simulink subsystem "BAM_Controller"  (R2026a)
settings: Solver=VariableStepAuto
undefined symbols (not defined in the file): DiscIntNeverNeededParam, SimIn, SimPar
libraries: simulink x11, starslibMathOperations x2, sharedTrackingLibrary x1, simulink_extras x1, starslibAxisTransformations x1
(part 1 of 3)
settings Model: Creator=macheson  LastModifiedBy=wyatt

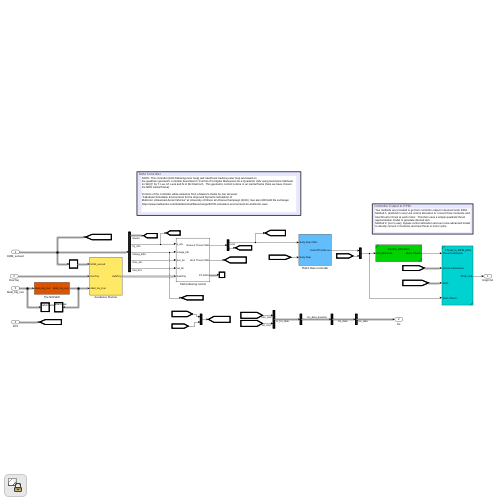
[thumbnail: Simulink's stored preview of the top-level diagram]
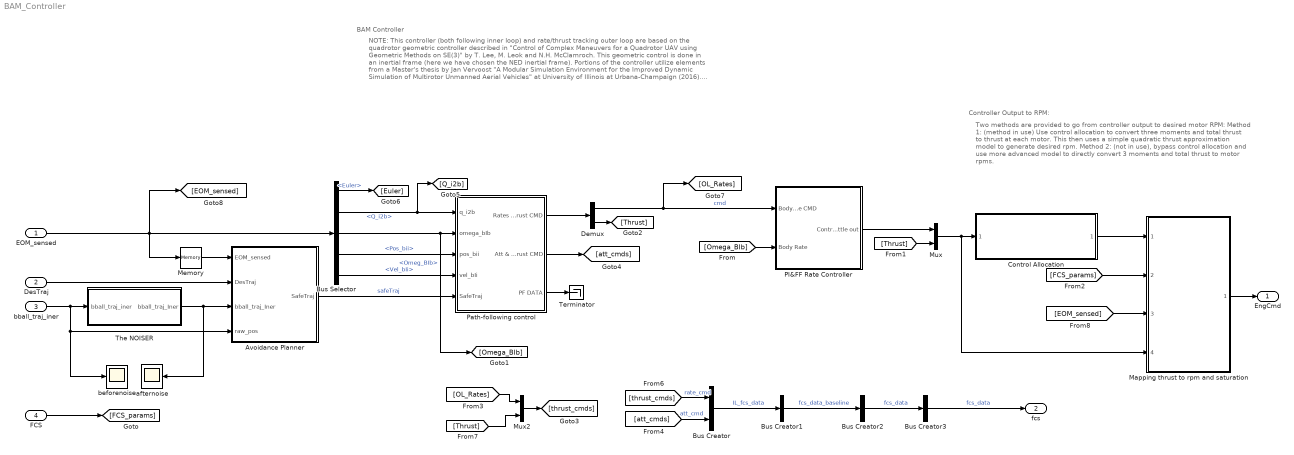
== system BAM_Controller ==
  note: NOTE: This controller (both following inner loop) and rate/thrust tracking outer loop are based on
      | the quadrotor geometric controller described in "Control of Complex Maneuvers for a Quadrotor UAV using Geometric Methods on SE(3)" by T. Lee, M. Leok and N.H. McClamroch. This geometric control is done in an inertial frame (here we have chosen the NED inertial frame).
      |
      | Portions of the controller utilize elements from a Master's thesis by Jan Vervoost
      | "A Modular Simulation Environment for the Improved Dynamic Simulation of
      | Multirotor Unmanned Aerial Vehicles" at University of Illinois at Urbana-Champaign (2016). See also MATLAB file exchange:
      | https://www.mathworks.com/matlabcentral/fileexchange/59705-simulation-environment-for-multirotor-uavs
  note: BAM Controller
  note: Controller Output to RPM:
  note: Two methods are provided to go from controller output to desired motor RPM:
      | Method 1: (method in use) Use control allocation to convert three moments and total thrust to thrust at each motor. This then uses a simple quadratic thrust approximation model to generate desired rpm.
      | Method 2: (not in use), bypass control allocation and use more advanced model to directly convert 3 moments and total thrust to motor rpms.
  EOM_sensed : Inport
  DesTraj : Inport  Port=2
  bball_traj_iner : Inport  Port=3
  FCS : Inport  Port=4
  Avoidance Planner : Subsystem
  Bus Creator : BusCreator  Inputs=2
  Bus Creator1 : BusCreator  Inputs=1
  Bus Creator2 : BusCreator  Inputs=1
  Bus Creator3 : BusCreator  Inputs=1
  Bus Selector : BusSelector  OutputSignals=WorldRelativeData.Euler,InertialData.Q_i2b,InertialData.Omeg_BIb,InertialData.Pos_bii,InertialData.Vel_bIi
  Control Allocation : Subsystem  ReferencedSubsystem=Control_Allocation
  Demux : Demux  Outputs=[3 1]
  Mapping thrust to rpm and saturation : Subsystem  ReferencedSubsystem=Thrust_to_RPM_MDL
  Memory : Memory
  Mux : Mux  Inputs=2
  Mux2 : Mux  Inputs=2
  PI&FF Rate Controller : Subsystem
  Path-following control : Subsystem
  Terminator : Terminator
  The NOISER : Subsystem
  afternoise : Scope
      settings: ActiveDisplayYMinimum=-1  ActiveDisplayYMaximum=1  DataLoggingVariableName=ScopeData14
  beforenoise : Scope
      settings: ActiveDisplayYMinimum=-48.7860252359001  ActiveDisplayYMaximum=146.64274370042804  DataLoggingVariableName=ScopeData15
  EngCmd : Outport  VectorParamsAs1DForOutWhenUnconnected=off
  fcs : Outport  Port=2  VectorParamsAs1DForOutWhenUnconnected=off
  wires:
  Path-following control/1(Rates & Thrust CMD) -> Demux/1
  [FCS_params] -> Mapping thrust to rpm and saturation/2
  Path-following control/3(PF DATA) -> Terminator/1
  EOM_sensed/1 -> [EOM_sensed], Bus Selector/1, Memory/1
  FCS/1 -> [FCS_params]
  PI&FF Rate Controller/1(Control/Throttle out) -> Mux/1
  Bus Selector/2 -> Path-following control/1(q_i2b), [Q_i2b]  "<Q_i2b>"
  Bus Selector/5 -> Path-following control/4(vel_bIi)  "<Vel_bIi>"
  Bus Selector/4 -> Path-following control/3(pos_bii)  "<Pos_bii>"
  Bus Selector/3 -> Path-following control/2(omega_bIb), [Omega_BIb]  "<Omeg_BIb>"
  [Omega_BIb] -> PI&FF Rate Controller/2(Body Rate)
  Demux/2 -> [Thrust]
  Demux/1 -> PI&FF Rate Controller/1(Body Rate CMD), [OL_Rates]  "cmd"
  DesTraj/1 -> Avoidance Planner/2(DesTraj)
  Bus Creator/1 -> Bus Creator1/1  "IL_fcs_data"
  Bus Creator1/1 -> Bus Creator2/1  "fcs_data_baseline"
  Bus Creator2/1 -> Bus Creator3/1  "fcs_data"
  Bus Creator3/1 -> fcs/1  "fcs_data"
  Path-following control/2(Att & Thrust CMD) -> [att_cmds]
  Bus Selector/1 -> [Euler]  "<Euler>"
  [thrust_cmds] -> Bus Creator/1  "rate_cmd"
  Mux2/1 -> [thrust_cmds]
  [OL_Rates] -> Mux2/1
  [Thrust] -> Mux2/2
  [Thrust] -> Mux/2
  Mux/1 -> Control Allocation/1, Mapping thrust to rpm and saturation/4
  Mapping thrust to rpm and saturation/1 -> EngCmd/1
  [att_cmds] -> Bus Creator/2  "att_cmd"
  [EOM_sensed] -> Mapping thrust to rpm and saturation/3
  Control Allocation/1 -> Mapping thrust to rpm and saturation/1
  Avoidance Planner/1(SafeTraj) -> Path-following control/5(SafeTraj)  "safeTraj"
  Memory/1 -> Avoidance Planner/1(EOM_sensed)
  bball_traj_iner/1 -> The NOISER/1(bball_traj_iner), Avoidance Planner/4(raw_pos), beforenoise/1
  The NOISER/1(bball_traj_Iner) -> Avoidance Planner/3(bball_traj_Iner), afternoise/1

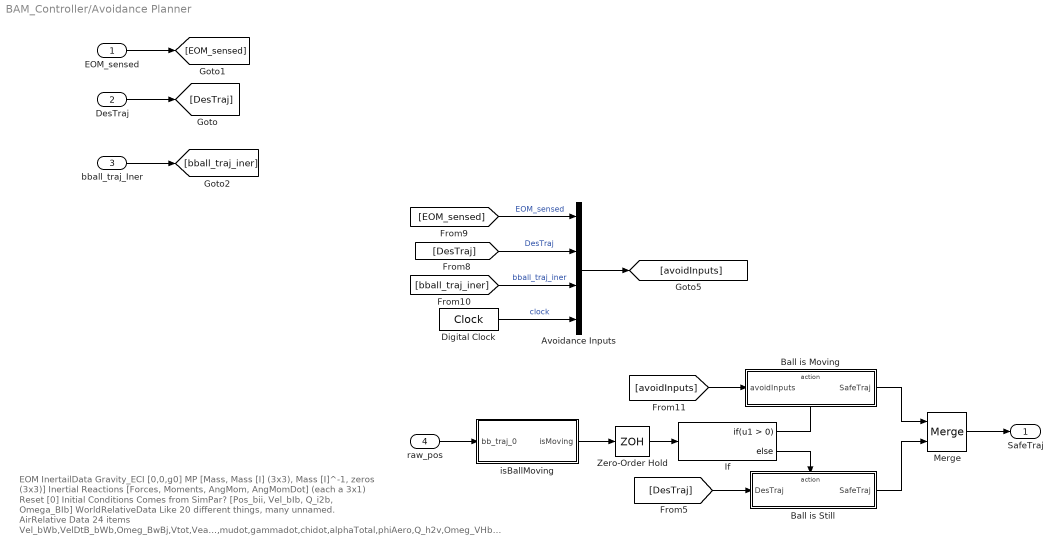
== system BAM_Controller/Avoidance Planner ==
  note: EOM
      | InertailData
      | Gravity_ECI
      | [0,0,g0]
      | MP
      | [Mass, Mass [I] (3x3), Mass [I]^-1, zeros (3x3)]
      | Inertial Reactions
      | [Forces, Moments, AngMom, AngMomDot] (each a 3x1)
      | Reset [0]
      | Initial Conditions
      | Comes from SimPar?
      | [Pos_bii, Vel_bIb, Q_i2b, Omega_BIb]
      | WorldRelativeData
      | Like 20 different things, many unnamed.
      | AirRelative Data
      | 24 items
      | Vel_bWb,VelDtB_bWb,Omeg_BwBj,Vtot,Veas,Vcas,Mach,qbar,qc,alpha,beta,mu,gamma,chi,Vtotdot,alphadot,betadot,mudot,gammadot,chidot,alphaTotal,phiAero,Q_h2v,Omeg_VHb
      | WRD is built using Env and ID, ARD is buid from Env and WRD
      | Traj_Iner = DesTraj (Designated Trajectory)
      | SimPar.RefInputs.trajectory
      | [wptVect, timeVect, parseVect]
      | Bball_traj
      | [pos_i, vel_i, acc_i, chi_des, chi_dot_des, time_violate_flag]
      | [(3,1), (3,1), (3,1), 1, 1, 1]
  EOM_sensed : Inport
  DesTraj : Inport  Port=2
  bball_traj_Iner : Inport  Port=3
  raw_pos : Inport  Port=4
  Avoidance Inputs : BusCreator  Inputs=4
  Ball is Moving : Subsystem  TreatAsAtomicUnit=on
  Ball is Still : Subsystem  TreatAsAtomicUnit=on
  Digital Clock : DigitalClock  SampleTime=.005
  If : If
  Merge : Merge
  Zero-Order Hold : ZeroOrderHold  SampleTime=.005
  isBallMoving : Subsystem
  SafeTraj : Outport
  wires:
  Digital Clock/1 -> Avoidance Inputs/4  "clock"
  isBallMoving/1(isMoving) -> Zero-Order Hold/1
  Avoidance Inputs/1 -> [avoidInputs]
  [bball_traj_iner] -> Avoidance Inputs/3  "bball_traj_iner"
  [DesTraj] -> Avoidance Inputs/2  "DesTraj"
  [EOM_sensed] -> Avoidance Inputs/1  "EOM_sensed"
  bball_traj_Iner/1 -> [bball_traj_iner]
  EOM_sensed/1 -> [EOM_sensed]
  DesTraj/1 -> [DesTraj]
  If/1 -> Ball is Moving/Action
  [avoidInputs] -> Ball is Moving/1(avoidInputs)
  Zero-Order Hold/1 -> If/1
  Ball is Moving/1(SafeTraj) -> Merge/1
  [DesTraj] -> Ball is Still/1(DesTraj)
  raw_pos/1 -> isBallMoving/1(bb_traj_0)
  If/2 -> Ball is Still/Action
  Merge/1 -> SafeTraj/1
  Ball is Still/1(SafeTraj) -> Merge/2

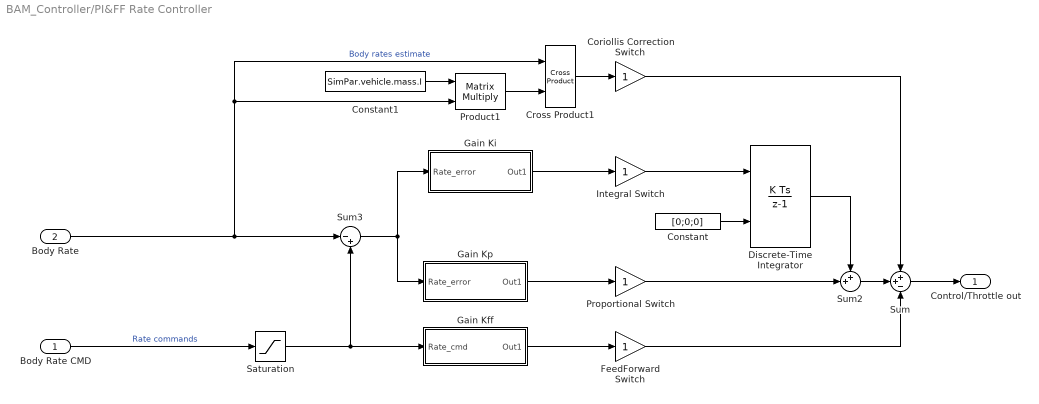
== system BAM_Controller/PI&FF Rate Controller ==
  Body Rate CMD : Inport
  Body Rate : Inport  Port=2
  Constant : Constant  Value=[0;0;0]  VectorParams1D=off
  Constant1 : Constant  Value=SimPar.vehicle.mass.I
  Coriollis Correction Switch : Gain
  Cross Product1 : starslibMathOperations/Cross Product
  Discrete-Time Integrator : DiscreteIntegrator  InitialConditionSource=external  SampleTime=SimIn.FCS.t_control  LimitOutput=on  UpperSaturationLimit=0.05  LowerSaturationLimit=-0.05  ICPrevOutput=DiscIntNeverNeededParam  ICPrevScaledInput=DiscIntNeverNeededParam
  FeedForward Switch : Gain
  Gain Kff : Subsystem
  Gain Ki : Subsystem
  Gain Kp : Subsystem
  Integral Switch : Gain
  Product1 : Product  Multiplication=Matrix(*)  RndMeth=Zero
  Proportional Switch : Gain
  Saturation : Saturate  UpperLimit=SimIn.FCS.maxRateCmd(3)  LowerLimit=-SimIn.FCS.maxRateCmd(3)
  Sum : Sum  Inputs=++-
  Sum2 : Sum  Inputs=++|
  Sum3 : Sum  Inputs=|-+
  Control/Throttle out : Outport  VectorParamsAs1DForOutWhenUnconnected=off
  wires:
  Coriollis Correction Switch/1 -> Sum/1
  Cross Product1/1 -> Coriollis Correction Switch/1
  Body Rate/1 -> Sum3/1, Product1/2, Cross Product1/1  "Body rates estimate"
  Constant1/1 -> Product1/1
  Product1/1 -> Cross Product1/2
  FeedForward Switch/1 -> Sum/3
  Proportional Switch/1 -> Sum2/2
  Integral Switch/1 -> Discrete-Time Integrator/1
  Constant/1 -> Discrete-Time Integrator/2
  Gain Ki/1(Out1) -> Integral Switch/1
  Saturation/1 -> Sum3/2, Gain Kff/1(Rate_cmd)
  Gain Kff/1(Out1) -> FeedForward Switch/1
  Sum2/1 -> Sum/2
  Sum3/1 -> Gain Kp/1(Rate_error), Gain Ki/1(Rate_error)
  Body Rate CMD/1 -> Saturation/1  "Rate commands"
  Sum/1 -> Control/Throttle out/1
  Gain Kp/1(Out1) -> Proportional Switch/1
  Discrete-Time Integrator/1 -> Sum2/1

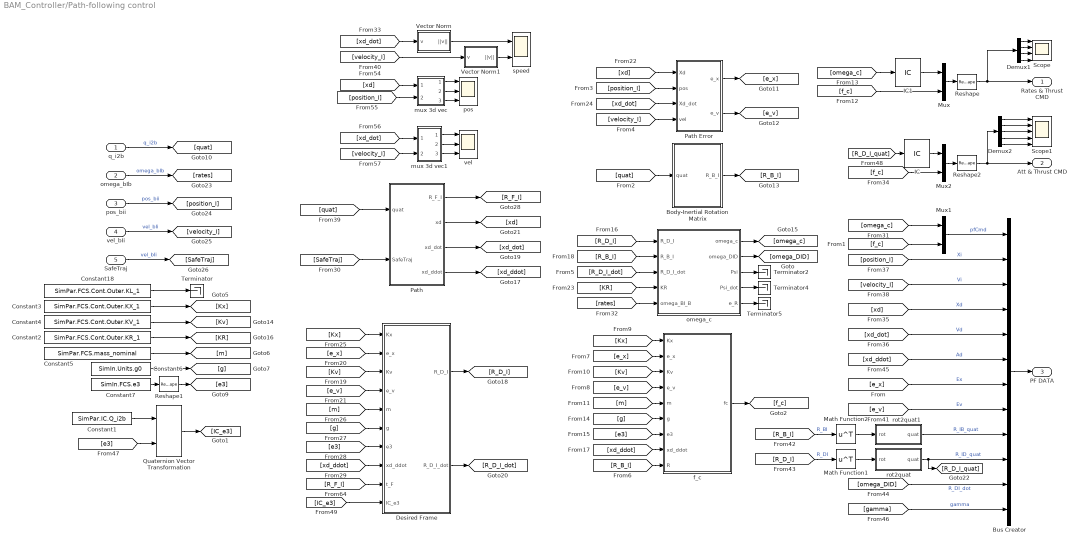
== system BAM_Controller/Path-following control ==
  q_i2b : Inport
  omega_bIb : Inport  Port=2
  pos_bii : Inport  Port=3
  vel_bIi : Inport  Port=4
  SafeTraj : Inport  Port=5
  Body-Inertial Rotation Matrix : Subsystem
  Bus Creator : BusCreator  Inputs=12
  Constant1 : Constant  Value=SimPar.IC.Q_i2b  VectorParams1D=off
  Constant18 : Constant  Value=SimPar.FCS.Cont.Outer.KL_1
  Constant2 : Constant  Value=SimPar.FCS.Cont.Outer.KR_1
  Constant3 : Constant  Value=SimPar.FCS.Cont.Outer.KX_1
  Constant4 : Constant  Value=SimPar.FCS.Cont.Outer.KV_1
  Constant5 : Constant  Value=SimPar.FCS.mass_nominal
  Constant6 : Constant  Value=SimIn.Units.g0
  Constant7 : Constant  Value=SimIn.FCS.e3  VectorParams1D=off
  Demux1 : Demux
  Demux2 : Demux  Outputs=5
  Desired Frame : Subsystem
  IC : InitialCondition  Value=SimIn.IC.Q_i2b
  IC1 : InitialCondition  Value=SimIn.IC.Omega_BIb
  Math Function1 : Math  Operator=transpose  SignedPower=on
  Math Function2 : Math  Operator=transpose  SignedPower=on
  Mux : Mux  Inputs=2
  Mux1 : Mux  Inputs=2
  Mux2 : Mux  Inputs=2
  Path : Subsystem
  Path Error : Subsystem
  Quaternion Vector Transformation : starslibAxisTransformations/Quaternion Vector Transformation  n=0
  Reshape : Reshape  OutputDimensionality=Column vector (2-D)
  Reshape1 : Reshape  OutputDimensionality=Column vector (2-D)
  Reshape2 : Reshape  OutputDimensionality=Column vector (2-D)
  Scope : Scope  NumInputPorts=4
      settings: SampleTime=SimIn.model_params.sim_rate  ActiveDisplayYMinimum=-0.00169  ActiveDisplayYMaximum=0.00216
  Scope1 : Scope  NumInputPorts=5
      settings: SampleTime=SimIn.model_params.sim_rate  ActiveDisplayYMinimum=-0.00169  ActiveDisplayYMaximum=0.00216
  Terminator{,2,4..5} (4 alike) : Terminator
  Vector Norm : Subsystem  mask(Vector Norm){}
      mask help: Calculates the 2-norm of the input vector.
      settings: CopyFcn=set_param(gcb,'LinkStatus','none')
  Vector Norm1 : Subsystem  mask(Vector Norm){}
      mask help: Calculates the 2-norm of the input vector.
      settings: CopyFcn=set_param(gcb,'LinkStatus','none')
  f_c : Subsystem
  mux 3d vec : Subsystem
  mux 3d vec1 : Subsystem
  omega_c : Subsystem
  pos : Scope  NumInputPorts=3
      settings: SampleTime=SimIn.model_params.sim_rate  ActiveDisplayYMinimum=-7386.0314  ActiveDisplayYMaximum=820.67244  DataLoggingVariableName=ScopeData2
  rot2quat : Subsystem  mask(RotationMatrix2Quat){}
      mask help: Rotation matrix to quaternion conversion.
      settings: CopyFcn=set_param(gcb,'LinkStatus','none')
  rot2quat1 : Subsystem  mask(RotationMatrix2Quat){}
      mask help: Rotation matrix to quaternion conversion.
      settings: CopyFcn=set_param(gcb,'LinkStatus','none')
  speed : Scope  NumInputPorts=2
      settings: SampleTime=SimIn.model_params.sim_rate  ActiveDisplayYMinimum=-0.50184  ActiveDisplayYMaximum=4.51655
  vel : Scope  NumInputPorts=3
      settings: SampleTime=SimIn.model_params.sim_rate  ActiveDisplayYMinimum=-3E-12  ActiveDisplayYMaximum=2.5E-11  DataLoggingVariableName=ScopeData3
  Rates & Thrust CMD : Outport  VectorParamsAs1DForOutWhenUnconnected=off
  Att & Thrust CMD : Outport  Port=2  VectorParamsAs1DForOutWhenUnconnected=off
  PF DATA : Outport  Port=3  VectorParamsAs1DForOutWhenUnconnected=off
  wires:
  IC/1 -> Mux2/1
  IC1/1 -> Mux/1
  [omega_c] -> IC1/1
  [R_D_I_quat] -> IC/1
  Demux2/5 -> Scope1/5
  [f_c] -> Mux2/2
  Demux2/2 -> Scope1/2
  Demux2/4 -> Scope1/4
  Reshape2/1 -> Demux2/1, Att & Thrust CMD/1
  Mux2/1 -> Reshape2/1
  Demux2/3 -> Scope1/3
  Demux2/1 -> Scope1/1
  [SafeTraj] -> Path/2(SafeTraj)
  SafeTraj/1 -> [SafeTraj]  "vel_bIi"
  vel_bIi/1 -> [velocity_I]  "vel_bIi"
  pos_bii/1 -> [position_I]  "pos_bii"
  omega_bIb/1 -> [rates]  "omega_bIb"
  [velocity_I] -> Vector Norm1/1(v)
  Vector Norm1/1(||v||) -> speed/2
  Vector Norm/1(||v||) -> speed/1
  [xd_dot] -> Vector Norm/1(v)
  rot2quat1/1(quat) -> Bus Creator/9  "R_IB_quat"
  Math Function2/1 -> rot2quat1/1(rot)
  omega_c/2(omega_DID) -> [omega_DID]
  [R_D_I] -> Math Function1/1  "R_DI"
  Math Function1/1 -> rot2quat/1(rot)
  Bus Creator/1 -> PF DATA/1
  [gamma] -> Bus Creator/12  "gamma"
  [omega_DID] -> Bus Creator/11  "R_DI_dot"
  rot2quat/1(quat) -> Bus Creator/10, [R_D_I_quat]  "R_ID_quat"
  [R_B_I] -> Math Function2/1  "R_BI"
  [e_v] -> Bus Creator/8  "Ev"
  [e_x] -> Bus Creator/7  "Ex"
  [xd_ddot] -> Bus Creator/6  "Ad"
  [xd_dot] -> Bus Creator/5  "Vd"
  [xd] -> Bus Creator/4  "Xd"
  [velocity_I] -> Bus Creator/3  "Vi"
  [position_I] -> Bus Creator/2  "Xi"
  [omega_c] -> Mux1/1
  Mux1/1 -> Bus Creator/1  "pfCmd"
  [f_c] -> Mux1/2
  [quat] -> Path/1(quat)
  f_c/1(fc) -> [f_c]
  [R_B_I] -> f_c/9(R)
  [xd_ddot] -> f_c/8(xd_ddot)
  [e3] -> f_c/7(e3)
  [g] -> f_c/6(g)
  [m] -> f_c/5(m)
  [e_v] -> f_c/4(e_v)
  [Kv] -> f_c/3(Kv)
  [e_x] -> f_c/2(e_x)
  [Kx] -> f_c/1(Kx)
  omega_c/1(omega_c) -> [omega_c]
  omega_c/5(e_R) -> Terminator5/1
  omega_c/4(Psi_dot) -> Terminator4/1
  omega_c/3(Psi) -> Terminator2/1
  [rates] -> omega_c/5(omega_BI_B)
  [KR] -> omega_c/4(KR)
  [R_D_I_dot] -> omega_c/3(R_D_I_dot)
  [R_B_I] -> omega_c/2(R_B_I)
  [R_D_I] -> omega_c/1(R_D_I)
  Desired Frame/2(R_D_I_dot) -> [R_D_I_dot]
  Desired Frame/1(R_D_I) -> [R_D_I]
  Path/1(R_F_I) -> [R_F_I]
  Path/4(xd_ddot) -> [xd_ddot]
  Path/3(xd_dot) -> [xd_dot]
  Path/2(xd) -> [xd]
  [velocity_I] -> mux 3d vec1/2(In2)
  [xd_dot] -> mux 3d vec1/1(In1)
  mux 3d vec1/3(Out3) -> vel/3
  mux 3d vec1/2(Out2) -> vel/2
  mux 3d vec1/1(Out1) -> vel/1
  [position_I] -> mux 3d vec/2(In2)
  [xd] -> mux 3d vec/1(In1)
  mux 3d vec/3(Out3) -> pos/3
  mux 3d vec/2(Out2) -> pos/2
  mux 3d vec/1(Out1) -> pos/1
  Reshape1/1 -> [e3]
  Constant6/1 -> [g]
  Constant5/1 -> [m]
  Constant7/1 -> Reshape1/1
  Constant2/1 -> [KR]
  Constant4/1 -> [Kv]
  Constant3/1 -> [Kx]
  Constant18/1 -> Terminator/1
  Body-Inertial Rotation Matrix/1(R_B_I) -> [R_B_I]
  [quat] -> Body-Inertial Rotation Matrix/1(quat)
  Reshape/1 -> Demux1/1, Rates & Thrust CMD/1
  Demux1/4 -> Scope/4
  Demux1/3 -> Scope/3
  Demux1/2 -> Scope/2
  Demux1/1 -> Scope/1
  Mux/1 -> Reshape/1
  [f_c] -> Mux/2
  [xd_dot] -> Path Error/3(Xd_dot)
  [xd] -> Path Error/1(Xd)
  Path Error/2(e_v) -> [e_v]
  Path Error/1(e_x) -> [e_x]
  [velocity_I] -> Path Error/4(vel)
  [position_I] -> Path Error/2(pos)
  q_i2b/1 -> [quat]  "q_i2b"
  [Kx] -> Desired Frame/1(Kx)
  [e_x] -> Desired Frame/2(e_x)
  [Kv] -> Desired Frame/3(Kv)
  [e_v] -> Desired Frame/4(e_v)
  [m] -> Desired Frame/5(m)
  [g] -> Desired Frame/6(g)
  [e3] -> Desired Frame/7(e3)
  [xd_ddot] -> Desired Frame/8(xd_ddot)
  [R_F_I] -> Desired Frame/9(t_F)
  Constant1/1 -> Quaternion Vector Transformation/1
  [IC_e3] -> Desired Frame/10(IC_e3)
  [e3] -> Quaternion Vector Transformation/2
  Quaternion Vector Transformation/1 -> [IC_e3]

== system BAM_Controller/The NOISER ==
  note: 0 = no noise
      | 0.1 = 10% noise
      | 0.5 = 50% noise
  bball_traj_iner : Inport
  Band-Limited White Noise : simulink/Sources/Band-Limited White Noise  Cov=[0]  Ts=0.1  seed=[23341]
  Bus Creator : BusCreator  Inputs=6  OutDataTypeStr=Bus: BUS_REF_INPUT_INER
  Bus Selector1 : BusSelector  OutputSignals=pos_i,vel_i,acc_i,chi_des,chi_dot_des,time_violate_flag
  Sum5 : Sum  Inputs=++|
  bball_traj_Iner : Outport
  wires:
  Band-Limited White Noise/1 -> Sum5/1
  Bus Selector1/1 -> Sum5/2  "<pos_i>"
  Bus Creator/1 -> bball_traj_Iner/1
  Sum5/1 -> Bus Creator/1  "pos_i"
  Bus Selector1/2 -> Bus Creator/2  "<vel_i>"
  Bus Selector1/3 -> Bus Creator/3  "<acc_i>"
  Bus Selector1/4 -> Bus Creator/4  "<chi_des>"
  Bus Selector1/5 -> Bus Creator/5  "<chi_dot_des>"
  Bus Selector1/6 -> Bus Creator/6  "<time_violate_flag>"
  bball_traj_iner/1 -> Bus Selector1/1

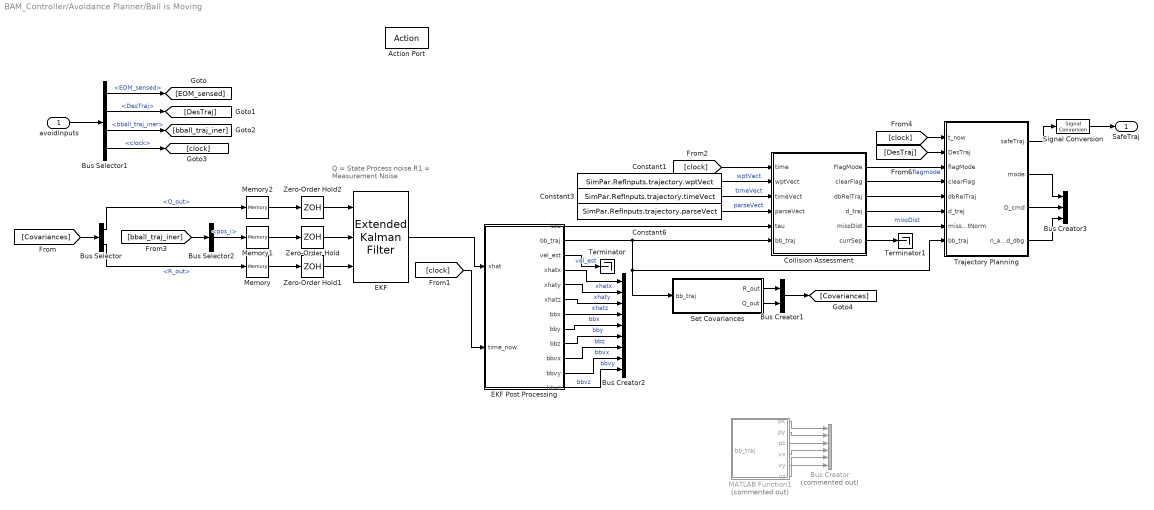
== system BAM_Controller/Avoidance Planner/Ball is Moving ==
  note: Q = State Process noise
      | R1 = Measurement Noise
  avoidInputs : Inport
  Action Port : ActionPort
  Bus Creator : BusCreator  Commented=on  Inputs=6
  Bus Creator1 : BusCreator  Inputs=2
  Bus Creator2 : BusCreator  Inputs=9
  Bus Creator3 : BusCreator  Inputs=3
  Bus Selector : BusSelector  OutputSignals=Q_out,R_out
  Bus Selector1 : BusSelector  OutputSignals=EOM_sensed,DesTraj,bball_traj_iner,clock
  Bus Selector2 : BusSelector  OutputSignals=pos_i
  Collision Assessment : MATLAB Function  TreatAsAtomicUnit=on
  Constant1 : Constant  Value=SimPar.RefInputs.trajectory.wptVect
  Constant3 : Constant  Value=SimPar.RefInputs.trajectory.timeVect
  Constant6 : Constant  Value=SimPar.RefInputs.trajectory.parseVect
  EKF : sharedTrackingLibrary/Extended Kalman Filter  StateTransitionFcn=ballStateTransitionFcn  HasStateTransitionJacobianFcn=off  HasAdditiveProcessNoise=Additive  ProcessNoise=diag([0.01 0.01 0.01 0.1 0.1 0.1])  HasTimeVaryingProcessNoise=on  HasStateTransitionFcnExtraArgument=0  InitialState=[-4.55720896517794 90.7482900530603 -0.440339408827839 19.065442307483 8.77448054331578 -23.8809138575693]  InitialStateCovariance=diag([0, 0, 0, 0, 0, 0])  MeasurementFcn1=ballMeasurementFcn  HasMeasurementJacobianFcn1=off  HasMeasurementEnablePort1=off  HasAdditiveMeasurementNoise1=Additive  MeasurementNoise1=diag([0.1 0.1 0.1])  HasTimeVaryingMeasurementNoise1=on  HasMeasurementFcnExtraArgument1=0  HasMeasurementWrapping1=off  HasMeasurementJacobianFcn2=off  HasMeasurementEnablePort2=off  HasAdditiveMeasurementNoise2=Additive  MeasurementNoise2=1  HasTimeVaryingMeasurementNoise2=off  HasMeasurementFcnExtraArgument2=0  HasMeasurementWrapping2=off  HasMeasurementJacobianFcn3=off  HasMeasurementEnablePort3=off  HasAdditiveMeasurementNoise3=Additive  MeasurementNoise3=1  HasTimeVaryingMeasurementNoise3=off  HasMeasurementFcnExtraArgument3=0  HasMeasurementWrapping3=off  HasMeasurementJacobianFcn4=off  HasMeasurementEnablePort4=off  HasAdditiveMeasurementNoise4=Additive  MeasurementNoise4=1  HasTimeVaryingMeasurementNoise4=off  HasMeasurementFcnExtraArgument4=0  HasMeasurementWrapping4=off  HasMeasurementJacobianFcn5=off  HasMeasurementEnablePort5=off  HasAdditiveMeasurementNoise5=Additive  MeasurementNoise5=1  HasTimeVaryingMeasurementNoise5=off  HasMeasurementFcnExtraArgument5=0  HasMeasurementWrapping5=off  EnableMultirate=off  StateTransitionFcnSampleTime=1  MeasurementFcn1SampleTime=1  MeasurementFcn2SampleTime=1  MeasurementFcn3SampleTime=1  MeasurementFcn4SampleTime=1  MeasurementFcn5SampleTime=1  UseCurrentEstimator=on  OutputStateCovariance=off  DataType=double  SampleTime=.005  NumberOfMeasurements=1
  EKF Post Processing : MATLAB Function  TreatAsAtomicUnit=on
  MATLAB Function1 : MATLAB Function  Commented=on  TreatAsAtomicUnit=on
  Memory : Memory  InheritSampleTime=on
  Memory1 : Memory  InheritSampleTime=on
  Memory2 : Memory  InheritSampleTime=on
  Set Covariances : MATLAB Function  TreatAsAtomicUnit=on
  Signal Conversion : SignalConversion  ConversionOutput=Virtual bus  OverrideOpt=off
  Terminator : Terminator
  Terminator1 : Terminator
  Trajectory Planning : MATLAB Function  TreatAsAtomicUnit=on
  Zero-Order Hold : ZeroOrderHold  SampleTime=.005
  Zero-Order Hold1 : ZeroOrderHold  SampleTime=.005
  Zero-Order Hold2 : ZeroOrderHold  SampleTime=.005
  SafeTraj : Outport
  wires:
  Collision Assessment/6(currSep) -> Terminator1/1
  Trajectory Planning/4(n_avoid_dbg) -> Bus Creator3/3
  Trajectory Planning/3(D_cmd) -> Bus Creator3/2
  Trajectory Planning/2(mode) -> Bus Creator3/1
  Collision Assessment/4(d_traj) -> Trajectory Planning/6(d_traj)
  [clock] -> Trajectory Planning/1(t_now)
  [clock] -> Collision Assessment/1(time)
  EKF Post Processing/12(bbvz) -> Bus Creator2/9  "bbvz"
  EKF Post Processing/4(xhatx) -> Bus Creator2/1  "xhatx"
  EKF Post Processing/5(xhaty) -> Bus Creator2/2  "xhaty"
  EKF Post Processing/6(xhatz) -> Bus Creator2/3  "xhatz"
  EKF Post Processing/7(bbx) -> Bus Creator2/4  "bbx"
  EKF Post Processing/8(bby) -> Bus Creator2/5  "bby"
  EKF Post Processing/9(bbz) -> Bus Creator2/6  "bbz"
  EKF Post Processing/10(bbvx) -> Bus Creator2/7  "bbvx"
  EKF Post Processing/11(bbvy) -> Bus Creator2/8  "bbvy"
  EKF Post Processing/3(vel_est) -> Terminator/1  "vel_est"
  Bus Selector1/4 -> [clock]  "<clock>"
  [clock] -> EKF Post Processing/2(time_now)
  MATLAB Function1/6(vz) -> Bus Creator/6
  MATLAB Function1/5(vy) -> Bus Creator/5
  MATLAB Function1/4(vx) -> Bus Creator/4
  MATLAB Function1/3(pz) -> Bus Creator/3
  MATLAB Function1/2(py) -> Bus Creator/2
  MATLAB Function1/1(px) -> Bus Creator/1
  Set Covariances/2(Q_out) -> Bus Creator1/2
  Set Covariances/1(R_out) -> Bus Creator1/1
  Signal Conversion/1 -> SafeTraj/1
  Bus Selector2/1 -> Memory1/1  "<pos_i>"
  [bball_traj_iner] -> Bus Selector2/1
  Bus Selector1/3 -> [bball_traj_iner]  "<bball_traj_iner>"
  Bus Selector1/2 -> [DesTraj]  "<DesTraj>"
  Bus Selector1/1 -> [EOM_sensed]  "<EOM_sensed>"
  avoidInputs/1 -> Bus Selector1/1
  Bus Selector/2 -> Memory/1  "<R_out>"
  [Covariances] -> Bus Selector/1
  Bus Creator1/1 -> [Covariances]
  EKF/1 -> EKF Post Processing/1(xhat)
  Zero-Order Hold/1 -> EKF/2
  Memory2/1 -> Zero-Order Hold2/1
  Bus Selector/1 -> Memory2/1  "<Q_out>"
  Zero-Order Hold2/1 -> EKF/1
  Zero-Order Hold1/1 -> EKF/3
  Memory/1 -> Zero-Order Hold1/1
  Memory1/1 -> Zero-Order Hold/1
  Trajectory Planning/1(safeTraj) -> Signal Conversion/1
  [DesTraj] -> Trajectory Planning/2(DesTraj)
  Collision Assessment/2(clearFlag) -> Trajectory Planning/4(clearFlag)
  Constant3/1 -> Collision Assessment/3(timeVect)  "timeVect"
  Collision Assessment/5(missDist) -> Trajectory Planning/7(missDistNorm)  "missDist"
  Collision Assessment/3(dbRelTraj) -> Trajectory Planning/5(dbRelTraj)
  EKF Post Processing/2(bb_traj) -> Collision Assessment/6(bb_traj), Trajectory Planning/8(bb_traj), Set Covariances/1(bb_traj)
  EKF Post Processing/1(tau) -> Collision Assessment/5(tau)
  Constant1/1 -> Collision Assessment/2(wptVect)  "wptVect"
  Collision Assessment/1(FlagMode) -> Trajectory Planning/3(flagMode)  "flagmode"
  Constant6/1 -> Collision Assessment/4(parseVect)  "parseVect"

== system BAM_Controller/Avoidance Planner/Ball is Still ==
  DesTraj : Inport
  Action Port : ActionPort
  SafeTraj : Outport
  wires:
  DesTraj/1 -> SafeTraj/1

== system BAM_Controller/Avoidance Planner/isBallMoving ==
  bb_traj_0 : Inport
  Bus Selector : BusSelector  OutputSignals=pos_i
  Compare To Constant : simulink/Logic and Bit Operations/Compare To Constant  relop=>  const=0.01  OutDataTypeStr=boolean
  Compare To Constant1 : simulink/Logic and Bit Operations/Compare To Constant  relop=>  const=0.01  OutDataTypeStr=boolean
  Constant7 : Constant  Value=1e-9
  Constant8 : Constant  Value=0
  Data Type Conversion2 : DataTypeConversion  OutDataTypeStr=boolean  SaturateOnIntegerOverflow=off  RndMeth=Floor
  Data Type Conversion3 : DataTypeConversion  OutDataTypeStr=boolean  SaturateOnIntegerOverflow=off  RndMeth=Floor
  Dot Product1 : DotProduct  OutDataTypeStr=Inherit: Inherit via internal rule
  S-R Flip-Flop1 : simulink_extras/Flip Flops/S-R Flip-Flop  initial_condition=0
  Sqrt1 : Sqrt
  Sum2 : Sum  Inputs=|+-
  Sum3 : Sum  Inputs=|++
  Unit Delay1 : UnitDelay  SampleTime=-1
  Zero-Order Hold2 : ZeroOrderHold  SampleTime=.005
  isMoving : Outport
  wires:
  Compare To Constant/1 -> Zero-Order Hold2/1
  Sqrt1/1 -> Compare To Constant/1
  Bus Selector/1 -> Unit Delay1/1, Sum2/1  "<pos_i>"
  bb_traj_0/1 -> Bus Selector/1
  Zero-Order Hold2/1 -> isMoving/1
  Sum3/1 -> Sqrt1/1
  Dot Product1/1 -> Sum3/1
  Unit Delay1/1 -> Sum2/2
  Sum2/1 -> Dot Product1/1, Dot Product1/2
  Constant8/1 -> Data Type Conversion3/1
  Constant7/1 -> Sum3/2
  Data Type Conversion3/1 -> S-R Flip-Flop1/2
  Data Type Conversion2/1 -> S-R Flip-Flop1/1
  Compare To Constant1/1 -> Data Type Conversion2/1

== system BAM_Controller/PI&FF Rate Controller/Gain Kff ==
  Rate_cmd : Inport
  Constant : Constant  Value=SimPar.vehicle.mass.I
  Constant1 : Constant  Value=SimPar.FCS.Cont.Inner.Kff_1
  Diagonalize Vector : Subsystem
  Product : Product  Multiplication=Matrix(*)  RndMeth=Zero
  Product1 : Product  Multiplication=Matrix(*)  RndMeth=Zero
  Out1 : Outport  VectorParamsAs1DForOutWhenUnconnected=off
  wires:
  Diagonalize Vector/1(Matrix) -> Product1/2
  Constant/1 -> Product1/1
  Product/1 -> Out1/1
  Constant1/1 -> Diagonalize Vector/1(Vector)
  Rate_cmd/1 -> Product/2
  Product1/1 -> Product/1

== system BAM_Controller/PI&FF Rate Controller/Gain Ki ==
  Rate_error : Inport
  Constant : Constant  Value=SimPar.vehicle.mass.I
  Constant1 : Constant  Value=SimPar.FCS.Cont.Inner.Ki_1
  Diagonalize Vector : Subsystem
  Product : Product  Multiplication=Matrix(*)  RndMeth=Zero
  Product1 : Product  Multiplication=Matrix(*)  RndMeth=Zero
  Out1 : Outport  VectorParamsAs1DForOutWhenUnconnected=off
  wires:
  Diagonalize Vector/1(Matrix) -> Product1/2
  Constant/1 -> Product1/1
  Product/1 -> Out1/1
  Constant1/1 -> Diagonalize Vector/1(Vector)
  Rate_error/1 -> Product/2
  Product1/1 -> Product/1

== system BAM_Controller/PI&FF Rate Controller/Gain Kp ==
  Rate_error : Inport
  Constant : Constant  Value=SimPar.vehicle.mass.I
  Constant1 : Constant  Value=SimPar.FCS.Cont.Inner.Kp_1
  Diagonalize Vector : Subsystem
  Product : Product  Multiplication=Matrix(*)  RndMeth=Zero
  Product1 : Product  Multiplication=Matrix(*)  RndMeth=Zero
  Out1 : Outport  VectorParamsAs1DForOutWhenUnconnected=off
  wires:
  Diagonalize Vector/1(Matrix) -> Product1/2
  Constant1/1 -> Diagonalize Vector/1(Vector)
  Constant/1 -> Product1/1
  Product/1 -> Out1/1
  Rate_error/1 -> Product/2
  Product1/1 -> Product/1

== system BAM_Controller/Path-following control/Body-Inertial Rotation Matrix ==
  quat : Inport
  MATLAB Function : MATLAB Function  TreatAsAtomicUnit=on
  Math Function6 : Math  Operator=transpose  SignedPower=on
  R_B_I : Outport  VectorParamsAs1DForOutWhenUnconnected=off
  wires:
  quat/1 -> MATLAB Function/1(q)
  MATLAB Function/1(R) -> Math Function6/1
  Math Function6/1 -> R_B_I/1

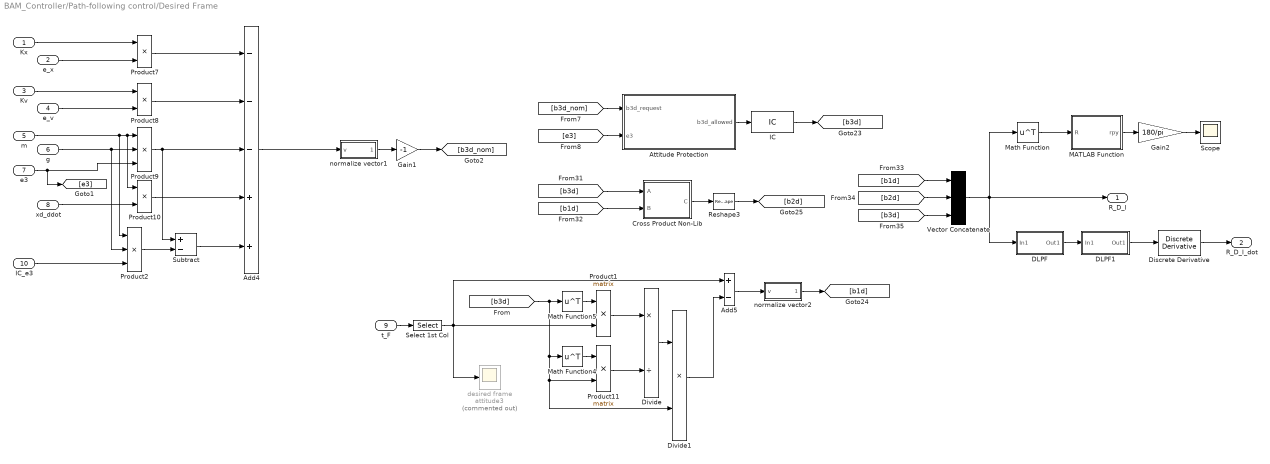
== system BAM_Controller/Path-following control/Desired Frame ==
  Kx : Inport
  e_x : Inport  Port=2
  Kv : Inport  Port=3
  e_v : Inport  Port=4
  m : Inport  Port=5
  g : Inport  Port=6
  e3 : Inport  Port=7
  xd_ddot : Inport  Port=8
  t_F : Inport  Port=9
  IC_e3 : Inport  Port=10
  Add4 : Sum  Inputs=---++
  Add5 : Sum  Inputs=+-
  Attitude Protection : Subsystem
  Cross Product Non-Lib : Subsystem
  DLPF : Subsystem  mask{w=20}
      mask prompts: w "Bandwidth"
      mask Display:
      | fprintf('%d rps',w)
      | port_label('input',  1, 'u')
      | port_label('output', 1, 'uf')
  DLPF1 : Subsystem  mask{w=20}
      mask prompts: w "Bandwidth"
      mask Display:
      | fprintf('%d rps',w)
      | port_label('input',  1, 'u')
      | port_label('output', 1, 'uf')
  Discrete Derivative : simulink/Discrete/Discrete Derivative  gainval=1.0  ICPrevScaledInput=0.0  OutMin=[]  OutMax=[]  OutDataType=fixdt(1, 16)  OutScaling=2^-10  DoSatur=off
  Divide : Product  Inputs=*/
  Divide1 : Product  Inputs=**
  Gain1 : Gain  Gain=-1
  Gain2 : Gain  Gain=180/pi
  IC : InitialCondition  Value=[0;0;1]
  MATLAB Function : MATLAB Function  TreatAsAtomicUnit=on
  Math Function : Math  Operator=transpose  SignedPower=on
  Math Function4 : Math  Operator=transpose  SignedPower=on
  Math Function5 : Math  Operator=transpose  SignedPower=on
  Product1 : Product  Multiplication=Matrix(*)
  Product10 : Product
  Product11 : Product  Multiplication=Matrix(*)
  Product2 : Product  Inputs=3
  Product7 : Product
  Product8 : Product
  Product9 : Product  Inputs=3
  Reshape3 : Reshape  OutputDimensionality=Column vector (2-D)
  Scope : Scope
  Select 1st Col : Selector  NumberOfDimensions=2  InputPortWidth=3  IndexOptions=Select all,Index vector (dialog)  Indices=[1 3],1  OutputSizes=1,1
  Subtract : Sum  Inputs=+-
  Vector Concatenate : Concatenate  NumInputs=3  Mode=Multidimensional array  ConcatenateDimension=2
  desired frame attitude3 : Scope  Commented=on
      settings: SampleTime=FCS.t_control  ActiveDisplayYMinimum=-0.67068  ActiveDisplayYMaximum=1.18563  DataLoggingVariableName=ScopeData2
  normalize vector1 : Subsystem
  normalize vector2 : Subsystem
  R_D_I : Outport  VectorParamsAs1DForOutWhenUnconnected=off
  R_D_I_dot : Outport  Port=2  VectorParamsAs1DForOutWhenUnconnected=off
  wires:
  Math Function/1 -> MATLAB Function/1(R)
  IC/1 -> [b3d]
  normalize vector2/1(v / ||v||) -> [b1d]
  Select 1st Col/1 -> Product1/2, Add5/1, desired frame attitude3/1
  Vector Concatenate/1 -> DLPF/1(In1), R_D_I/1, Math Function/1
  Attitude Protection/1(b3d_allowed) -> IC/1
  [e3] -> Attitude Protection/2(e3)
  [b3d_nom] -> Attitude Protection/1(b3d_request)
  Gain2/1 -> Scope/1
  MATLAB Function/1(rpy) -> Gain2/1
  DLPF1/1(Out1) -> Discrete Derivative/1
  DLPF/1(Out1) -> DLPF1/1(In1)
  Discrete Derivative/1 -> R_D_I_dot/1
  Product11/1 -> Divide/2
  Math Function5/1 -> Product1/1
  Divide/1 -> Divide1/1
  Divide1/1 -> Add5/2
  Product1/1 -> Divide/1
  Math Function4/1 -> Product11/1
  [b3d] -> Math Function5/1, Math Function4/1, Product11/2, Divide1/2
  t_F/1 -> Select 1st Col/1
  [b1d] -> Vector Concatenate/1
  [b3d] -> Vector Concatenate/3
  Cross Product Non-Lib/1(C) -> Reshape3/1
  [b1d] -> Cross Product Non-Lib/2(B)
  [b2d] -> Vector Concatenate/2
  [b3d] -> Cross Product Non-Lib/1(A)
  Reshape3/1 -> [b2d]
  Add5/1 -> normalize vector2/1(v)
  normalize vector1/1(v / ||v||) -> Gain1/1
  Add4/1 -> normalize vector1/1(v)
  Gain1/1 -> [b3d_nom]
  xd_ddot/1 -> Product10/2
  IC_e3/1 -> Product2/3
  Product2/1 -> Subtract/2
  e_x/1 -> Product7/2
  e3/1 -> [e3], Product9/3
  Product7/1 -> Add4/1
  Product9/1 -> Add4/3, Subtract/1
  Kv/1 -> Product8/1
  e_v/1 -> Product8/2
  Product10/1 -> Add4/4
  Kx/1 -> Product7/1
  m/1 -> Product9/1, Product10/1, Product2/1
  Subtract/1 -> Add4/5
  g/1 -> Product2/2, Product9/2
  Product8/1 -> Add4/2

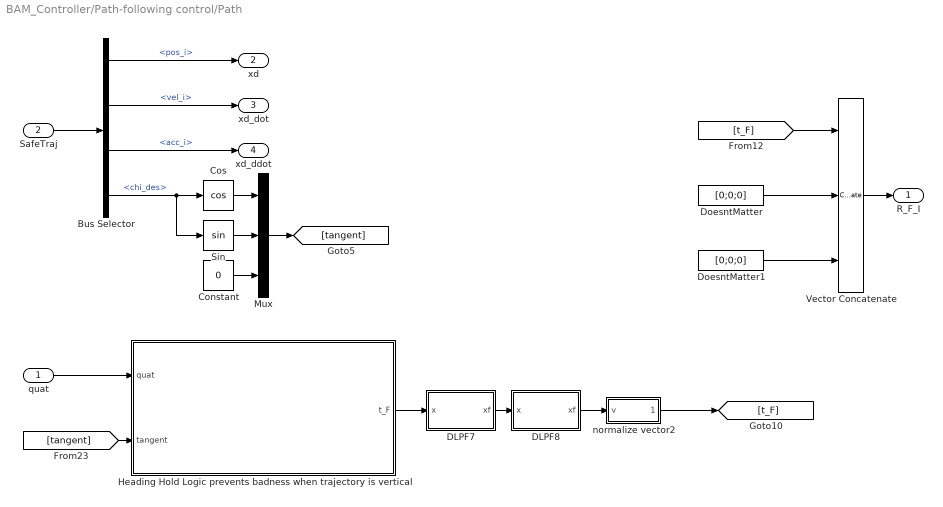
== system BAM_Controller/Path-following control/Path ==
  quat : Inport
  SafeTraj : Inport  Port=2
  Bus Selector : BusSelector  OutputSignals=pos_i,vel_i,acc_i,chi_des
  Constant : Constant  Value=0
  Cos : Trigonometry  Operator=cos
  DLPF7 : Subsystem  mask(Discrete Low-Pass Filter){bw=0.5}
      mask prompts: bw "Bandwidth"
      mask help: Low pass filter a signal with a discrete integrator. Initial condition is obtained from input.
      mask init:
      | set_param(gcb,'LinkStatus','none')
      settings: CopyFcn=set_param(gcb,'LinkStatus','none')
      mask Display:
      | port_label('input',1,'x');
      | port_label('output',1,'xf');
      | 
      | disp([get_param(gcb,'bw') ' rad/s']);
  DLPF8 : Subsystem  mask(Discrete Low-Pass Filter){bw=0.5}
      mask prompts: bw "Bandwidth"
      mask help: Low pass filter a signal with a discrete integrator. Initial condition is obtained from input.
      mask init:
      | set_param(gcb,'LinkStatus','none')
      settings: CopyFcn=set_param(gcb,'LinkStatus','none')
      mask Display:
      | port_label('input',1,'x');
      | port_label('output',1,'xf');
      | 
      | disp([get_param(gcb,'bw') ' rad/s']);
  DoesntMatter : Constant  Value=[0;0;0]  VectorParams1D=off
  DoesntMatter1 : Constant  Value=[0;0;0]  VectorParams1D=off
  Heading Hold Logic prevents badness when trajectory is vertical : Subsystem
  Mux : Mux  Inputs=3
  Sin : Trigonometry
  Vector Concatenate : Concatenate  NumInputs=3  Mode=Multidimensional array  ConcatenateDimension=2
  normalize vector2 : Subsystem
  R_F_I : Outport  VectorParamsAs1DForOutWhenUnconnected=off
  xd : Outport  Port=2  VectorParamsAs1DForOutWhenUnconnected=off
  xd_dot : Outport  Port=3  VectorParamsAs1DForOutWhenUnconnected=off
  xd_ddot : Outport  Port=4  VectorParamsAs1DForOutWhenUnconnected=off
  wires:
  Constant/1 -> Mux/3
  Sin/1 -> Mux/2
  Cos/1 -> Mux/1
  Bus Selector/4 -> Cos/1, Sin/1  "<chi_des>"
  Bus Selector/3 -> xd_ddot/1  "<acc_i>"
  Bus Selector/2 -> xd_dot/1  "<vel_i>"
  Bus Selector/1 -> xd/1  "<pos_i>"
  SafeTraj/1 -> Bus Selector/1
  normalize vector2/1(v / ||v||) -> [t_F]
  DLPF8/1(xf) -> normalize vector2/1(v)
  DLPF7/1(xf) -> DLPF8/1(x)
  Heading Hold Logic prevents badness when trajectory is vertical/1(t_F) -> DLPF7/1(x)
  [tangent] -> Heading Hold Logic prevents badness when trajectory is vertical/2(tangent)
  quat/1 -> Heading Hold Logic prevents badness when trajectory is vertical/1(quat)
  DoesntMatter1/1 -> Vector Concatenate/3
  DoesntMatter/1 -> Vector Concatenate/2
  Mux/1 -> [tangent]
  Vector Concatenate/1 -> R_F_I/1
  [t_F] -> Vector Concatenate/1

== system BAM_Controller/Path-following control/Path Error ==
  Xd : Inport
  pos : Inport  Port=2
  Xd_dot : Inport  Port=3
  vel : Inport  Port=4
  Add : Sum  Inputs=+-
  Add1 : Sum  Inputs=+-
  e_x : Outport  VectorParamsAs1DForOutWhenUnconnected=off
  e_v : Outport  Port=2  VectorParamsAs1DForOutWhenUnconnected=off
  wires:
  Xd_dot/1 -> Add1/2
  Xd/1 -> Add/2
  Add1/1 -> e_v/1
  Add/1 -> e_x/1
  pos/1 -> Add/1
  vel/1 -> Add1/1

== system BAM_Controller/Path-following control/Vector Norm ==
  v : Inport
  Math Function1 : Math  Operator=transpose  SignedPower=on
  Matrix Multiply1 : Product  Multiplication=Matrix(*)
  Reshape7 : Reshape  OutputDimensionality=Column vector (2-D)
  Sqrt3 : Sqrt
  ||v|| : Outport  VectorParamsAs1DForOutWhenUnconnected=off
  wires:
  Sqrt3/1 -> ||v||/1
  v/1 -> Reshape7/1
  Math Function1/1 -> Matrix Multiply1/1
  Matrix Multiply1/1 -> Sqrt3/1
  Reshape7/1 -> Matrix Multiply1/2, Math Function1/1

== system BAM_Controller/Path-following control/Vector Norm1 ==
  v : Inport
  Math Function1 : Math  Operator=transpose  SignedPower=on
  Matrix Multiply1 : Product  Multiplication=Matrix(*)
  Reshape7 : Reshape  OutputDimensionality=Column vector (2-D)
  Sqrt3 : Sqrt
  ||v|| : Outport  VectorParamsAs1DForOutWhenUnconnected=off
  wires:
  Reshape7/1 -> Math Function1/1, Matrix Multiply1/2
  Matrix Multiply1/1 -> Sqrt3/1
  Math Function1/1 -> Matrix Multiply1/1
  v/1 -> Reshape7/1
  Sqrt3/1 -> ||v||/1

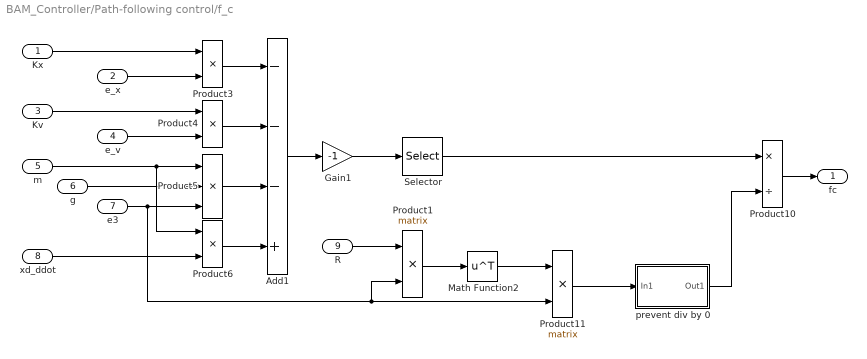
== system BAM_Controller/Path-following control/f_c ==
  Kx : Inport
  e_x : Inport  Port=2
  Kv : Inport  Port=3
  e_v : Inport  Port=4
  m : Inport  Port=5
  g : Inport  Port=6
  e3 : Inport  Port=7
  xd_ddot : Inport  Port=8
  R : Inport  Port=9
  Add1 : Sum  Inputs=---+
  Gain1 : Gain  Gain=-1
  Math Function2 : Math  Operator=transpose  SignedPower=on
  Product1 : Product  Multiplication=Matrix(*)
  Product10 : Product  Inputs=*/
  Product11 : Product  Multiplication=Matrix(*)
  Product3 : Product
  Product4 : Product
  Product5 : Product  Inputs=3
  Product6 : Product
  Selector : Selector  InputPortWidth=3  IndexOptions=Index vector (dialog)  Indices=[3]  OutputSizes=1
  prevent div by 0 : Subsystem
  fc : Outport  VectorParamsAs1DForOutWhenUnconnected=off
  wires:
  prevent div by 0/1(Out1) -> Product10/2
  Product11/1 -> prevent div by 0/1(In1)
  Selector/1 -> Product10/1
  Gain1/1 -> Selector/1
  Product10/1 -> fc/1
  Math Function2/1 -> Product11/1
  Add1/1 -> Gain1/1
  R/1 -> Product1/1
  e_x/1 -> Product3/2
  e_v/1 -> Product4/2
  e3/1 -> Product1/2, Product11/2, Product5/3
  Product1/1 -> Math Function2/1
  Kx/1 -> Product3/1
  Kv/1 -> Product4/1
  Product5/1 -> Add1/3
  Product3/1 -> Add1/1
  xd_ddot/1 -> Product6/2
  m/1 -> Product5/1, Product6/1
  Product6/1 -> Add1/4
  Product4/1 -> Add1/2
  g/1 -> Product5/2

== system BAM_Controller/Path-following control/mux 3d vec ==
  In1 : Inport
  In2 : Inport  Port=2
  Demux2 : Demux  Outputs=3
  Demux3 : Demux  Outputs=3
  Mux4 : Mux  Inputs=2
  Mux5 : Mux  Inputs=2
  Mux6 : Mux  Inputs=2
  Out1 : Outport  VectorParamsAs1DForOutWhenUnconnected=off
  Out2 : Outport  Port=2  VectorParamsAs1DForOutWhenUnconnected=off
  Out3 : Outport  Port=3  VectorParamsAs1DForOutWhenUnconnected=off
  wires:
  Demux2/2 -> Mux5/1
  Demux2/3 -> Mux6/1
  In1/1 -> Demux2/1
  In2/1 -> Demux3/1
  Mux6/1 -> Out3/1
  Mux5/1 -> Out2/1
  Mux4/1 -> Out1/1
  Demux3/3 -> Mux6/2
  Demux3/1 -> Mux4/2
  Demux3/2 -> Mux5/2
  Demux2/1 -> Mux4/1

== system BAM_Controller/Path-following control/mux 3d vec1 ==
  In1 : Inport
  In2 : Inport  Port=2
  Demux2 : Demux  Outputs=3
  Demux3 : Demux  Outputs=3
  Mux4 : Mux  Inputs=2
  Mux5 : Mux  Inputs=2
  Mux6 : Mux  Inputs=2
  Out1 : Outport  VectorParamsAs1DForOutWhenUnconnected=off
  Out2 : Outport  Port=2  VectorParamsAs1DForOutWhenUnconnected=off
  Out3 : Outport  Port=3  VectorParamsAs1DForOutWhenUnconnected=off
  wires:
  Demux2/1 -> Mux4/1
  Demux3/2 -> Mux5/2
  Demux3/1 -> Mux4/2
  Demux3/3 -> Mux6/2
  Mux4/1 -> Out1/1
  Mux5/1 -> Out2/1
  Mux6/1 -> Out3/1
  In2/1 -> Demux3/1
  In1/1 -> Demux2/1
  Demux2/3 -> Mux6/1
  Demux2/2 -> Mux5/1

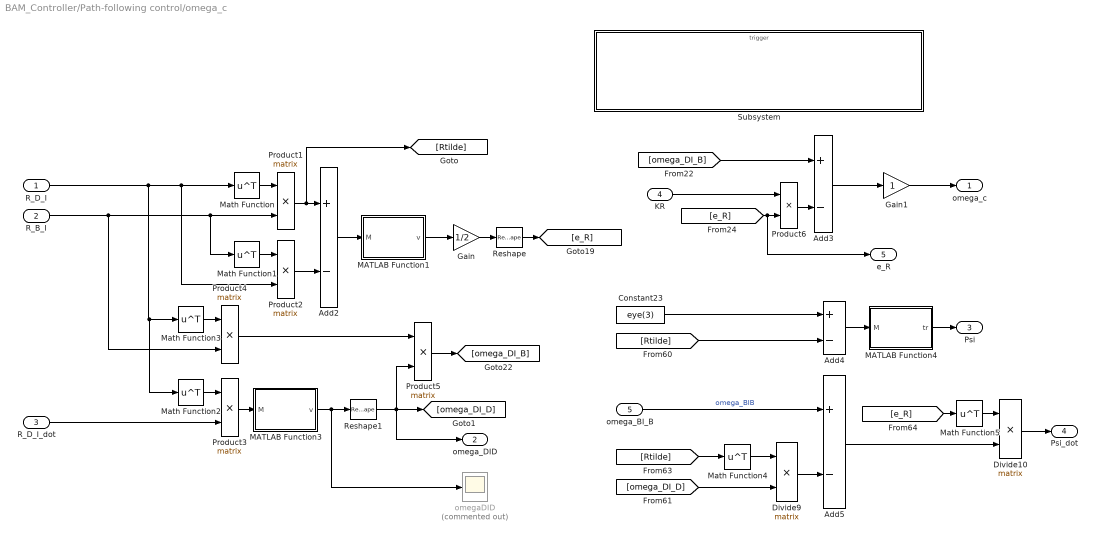
== system BAM_Controller/Path-following control/omega_c ==
  R_D_I : Inport
  R_B_I : Inport  Port=2
  R_D_I_dot : Inport  Port=3
  KR : Inport  Port=4
  omega_BI_B : Inport  Port=5
  Add{2..5} (4 alike) : Sum  Inputs=+-
  Constant23 : Constant  Value=eye(3)  VectorParams1D=off
  Divide10 : Product  Inputs=**  Multiplication=Matrix(*)
  Divide9 : Product  Inputs=**  Multiplication=Matrix(*)
  Gain : Gain  Gain=1/2
  Gain1 : Gain
  MATLAB Function1 : MATLAB Function  TreatAsAtomicUnit=on
  MATLAB Function3 : MATLAB Function  TreatAsAtomicUnit=on
  MATLAB Function4 : MATLAB Function  TreatAsAtomicUnit=on
  Math Function{,1..5} (6 alike) : Math  Operator=transpose  SignedPower=on
  Product{1..5} (5 alike) : Product  Multiplication=Matrix(*)
  Product6 : Product
  Reshape : Reshape  OutputDimensionality=Column vector (2-D)
  Reshape1 : Reshape  OutputDimensionality=Column vector (2-D)
  Subsystem : Subsystem
  omegaDID : Scope  Commented=on
      settings: SampleTime=FCS.t_control  ActiveDisplayYMinimum=-1.8E-6  ActiveDisplayYMaximum=1.4E-6  DataLoggingVariableName=ScopeData5
  omega_c : Outport  VectorParamsAs1DForOutWhenUnconnected=off
  omega_DID : Outport  Port=2  VectorParamsAs1DForOutWhenUnconnected=off
  Psi : Outport  Port=3  VectorParamsAs1DForOutWhenUnconnected=off
  Psi_dot : Outport  Port=4  VectorParamsAs1DForOutWhenUnconnected=off
  e_R : Outport  Port=5  VectorParamsAs1DForOutWhenUnconnected=off
  wires:
  Gain1/1 -> omega_c/1
  MATLAB Function3/1(v) -> Reshape1/1, omegaDID/1
  R_D_I/1 -> Math Function/1, Product2/2, Math Function3/1, Math Function2/1
  Reshape1/1 -> Product5/2, omega_DID/1, [omega_DI_D]
  Reshape/1 -> [e_R]
  Divide10/1 -> Psi_dot/1
  MATLAB Function4/1(tr) -> Psi/1
  Math Function5/1 -> Divide10/1
  [e_R] -> Math Function5/1
  Add5/1 -> Divide10/2
  omega_BI_B/1 -> Add5/1  "omega_BIB"
  Divide9/1 -> Add5/2
  Math Function4/1 -> Divide9/1
  [Rtilde] -> Math Function4/1
  [omega_DI_D] -> Divide9/2
  [Rtilde] -> Add4/2
  Constant23/1 -> Add4/1
  Add4/1 -> MATLAB Function4/1(M)
  Gain/1 -> Reshape/1
  MATLAB Function1/1(v) -> Gain/1
  Product5/1 -> [omega_DI_B]
  Add2/1 -> MATLAB Function1/1(M)
  R_D_I_dot/1 -> Product3/2
  Math Function2/1 -> Product3/1
  Product3/1 -> MATLAB Function3/1(M)
  Product1/1 -> Add2/1, [Rtilde]
  Math Function1/1 -> Product2/1
  Product6/1 -> Add3/2
  Add3/1 -> Gain1/1
  Product2/1 -> Add2/2
  Math Function/1 -> Product1/1
  Math Function3/1 -> Product4/1
  Product4/1 -> Product5/1
  KR/1 -> Product6/1
  R_B_I/1 -> Math Function1/1, Product1/2, Product4/2
  [e_R] -> Product6/2, e_R/1
  [omega_DI_B] -> Add3/1

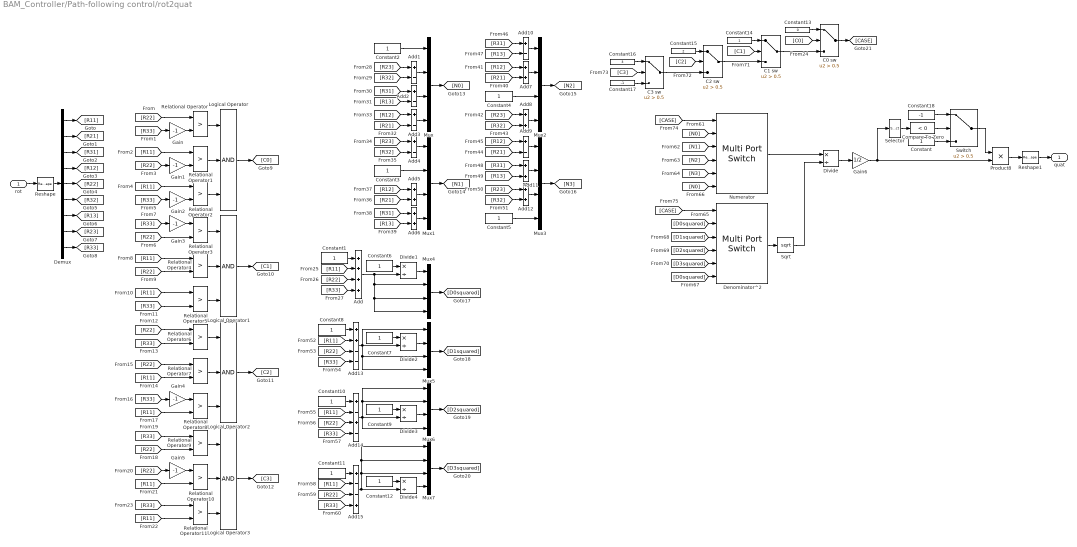
== system BAM_Controller/Path-following control/rot2quat ==
  rot : Inport
  Add : Sum  Inputs=++++
  Add{1..4,9..10} (6 alike) : Sum  Inputs=+-
  Add{5..8,11..12} (6 alike) : Sum
  Add13 : Sum  Inputs=++--
  Add14 : Sum  Inputs=+-+-
  Add15 : Sum  Inputs=+--+
  C0 sw : Switch  Criteria=u2 > Threshold  Threshold=0.5  SaturateOnIntegerOverflow=off  InputSameDT=off
  C1 sw : Switch  Criteria=u2 > Threshold  Threshold=0.5  SaturateOnIntegerOverflow=off  InputSameDT=off
  C2 sw : Switch  Criteria=u2 > Threshold  Threshold=0.5  SaturateOnIntegerOverflow=off  InputSameDT=off
  C3 sw : Switch  Criteria=u2 > Threshold  Threshold=0.5  SaturateOnIntegerOverflow=off  InputSameDT=off
  Compare To Zero : simulink/Logic and Bit Operations/Compare To Zero  relop=<  OutDataTypeStr=boolean
  Constant{,1..12,14} (14 alike) : Constant
  Constant13 : Constant  Value=0
  Constant15 : Constant  Value=2
  Constant16 : Constant  Value=3
  Constant17 : Constant  Value=-1
  Constant18 : Constant  Value=-1
  Demux : Demux  Outputs=9
  Denominator^2 : MultiPortSwitch  DataPortOrder=Zero-based contiguous  Inputs=4  DataPortForDefault=Additional data port  zeroidx=on  SaturateOnIntegerOverflow=off  InputSameDT=off
  Divide{,1..4} (5 alike) : Product  Inputs=*/
  Gain{,1..5} (6 alike) : Gain  Gain=-1
  Gain6 : Gain  Gain=1/2
  Logical Operator{,1..3} (4 alike) : Logic  Inputs=3  AllPortsSameDT=off  OutDataTypeStr=boolean
  Mux{,1..7} (8 alike) : Mux
  Numerator : MultiPortSwitch  DataPortOrder=Zero-based contiguous  Inputs=4  DataPortForDefault=Additional data port  zeroidx=on  SaturateOnIntegerOverflow=off  InputSameDT=off
  Product8 : Product
  Relational Operator{,1..11} (12 alike) : RelationalOperator  Operator=>  OutDataTypeStr=boolean  RndMeth=Simplest  InputSameDT=off
  Reshape : Reshape  OutputDimensionality=Column vector (2-D)
  Reshape1 : Reshape  OutputDimensionality=Column vector (2-D)
  Selector : Selector  InputPortWidth=4  IndexOptions=Index vector (dialog)  Indices=1  OutputSizes=1
  Sqrt : Sqrt
  Switch : Switch  Criteria=u2 > Threshold  Threshold=0.5  SaturateOnIntegerOverflow=off  InputSameDT=off
  quat : Outport  VectorParamsAs1DForOutWhenUnconnected=off
  wires:
  [R31] -> Add11/1
  Constant5/1 -> Mux3/4
  Constant1/1 -> Add/1
  [R23] -> Add8/1
  Add2/1 -> Mux/3
  Mux3/1 -> [N3]
  [R13] -> Add11/2
  Add11/1 -> Mux3/2
  Add8/1 -> Mux2/4
  [R32] -> Add8/2
  [R12] -> Add9/1
  Add9/1 -> Mux3/1
  Constant2/1 -> Mux/1
  Gain6/1 -> Product8/2, Selector/1
  [C1] -> C1 sw/2
  [R21] -> Add9/2
  Add13/1 -> Mux5/4, Mux5/3, Mux5/1, Divide2/2
  [D0squared] -> Denominator^2/6
  Mux5/1 -> [D1squared]
  Constant7/1 -> Divide2/1
  [N2] -> Numerator/4
  [R31] -> Add10/1
  [R31] -> Add2/1
  Add5/1 -> Mux1/3
  [C3] -> C3 sw/2
  [R21] -> Add5/2
  [R13] -> Add10/2
  Add10/1 -> Mux2/1
  C0 sw/1 -> [CASE]
  [R11] -> Add/2
  [R33] -> Add13/4
  Constant8/1 -> Add13/1
  Mux/1 -> [N0]
  [R32] -> Add1/2
  Constant10/1 -> Add14/1
  [R33] -> Add/4
  [R33] -> Add14/4
  [R22] -> Add13/3
  [R22] -> Add14/3
  Mux6/1 -> [D2squared]
  Add14/1 -> Mux6/1, Mux6/2, Mux6/4, Divide3/2
  Add1/1 -> Mux/2
  [R11] -> Add14/2
  [R11] -> Add13/2
  Constant9/1 -> Divide3/1
  [CASE] -> Numerator/1
  Add15/1 -> Mux7/1, Mux7/2, Mux7/3, Divide4/2
  Divide3/1 -> Mux6/3
  Constant15/1 -> C2 sw/1
  Constant16/1 -> C3 sw/1
  C3 sw/1 -> C2 sw/3
  [C2] -> C2 sw/2
  [C0] -> C0 sw/2
  Gain2/1 -> Relational Operator2/2
  Mux4/1 -> [D0squared]
  rot/1 -> Reshape/1
  [N1] -> Numerator/3
  [R31] -> Add6/1
  [R13] -> Add6/2
  Add3/1 -> Mux/4
  Add6/1 -> Mux1/4
  [R12] -> Add3/1
  Relational Operator7/1 -> Logical Operator2/2
  [R11] -> Relational Operator1/1
  Constant3/1 -> Mux1/2
  [R22] -> Add/3
  Constant12/1 -> Divide4/1
  [R22] -> Add15/3
  [R33] -> Add15/4
  Gain/1 -> Relational Operator/2
  [R22] -> Relational Operator7/1
  [R11] -> Relational Operator8/2
  [D3squared] -> Denominator^2/5
  Mux7/1 -> [D3squared]
  Logical Operator3/1 -> [C3]
  [R11] -> Relational Operator7/2
  Constant11/1 -> Add15/1
  Demux/7 -> [R13]
  Mux2/1 -> [N2]
  [R11] -> Add15/2
  [D1squared] -> Denominator^2/3
  Demux/9 -> [R33]
  [D0squared] -> Denominator^2/2
  Relational Operator6/1 -> Logical Operator2/1
  Add4/1 -> Mux1/1
  [CASE] -> Denominator^2/1
  [R23] -> Add4/1
  [R22] -> Gain1/1
  [R32] -> Add4/2
  [R22] -> Relational Operator6/1
  [R33] -> Relational Operator11/1
  [R33] -> Relational Operator6/2
  Logical Operator2/1 -> [C2]
  Logical Operator1/1 -> [C1]
  [R11] -> Relational Operator10/2
  [R33] -> Gain2/1
  [R22] -> Gain5/1
  Relational Operator11/1 -> Logical Operator3/3
  [R11] -> Relational Operator11/2
  Add12/1 -> Mux3/3
  Demux/2 -> [R21]
  Relational Operator3/1 -> Logical Operator1/1
  Demux/1 -> [R11]
  [R13] -> Add2/2
  Sqrt/1 -> Divide/2
  [R23] -> Add12/1
  [R32] -> Add12/2
  [D2squared] -> Denominator^2/4
  Constant4/1 -> Mux2/3
  Divide4/1 -> Mux7/4
  Constant13/1 -> C0 sw/1
  C1 sw/1 -> C0 sw/3
  Demux/8 -> [R23]
  Demux/5 -> [R22]
  [R33] -> Gain3/1
  Reshape/1 -> Demux/1
  Relational Operator1/1 -> Logical Operator/2
  Gain1/1 -> Relational Operator1/2
  [R22] -> Relational Operator3/2
  [R33] -> Gain4/1
  Relational Operator/1 -> Logical Operator/1
  [R11] -> Relational Operator2/1
  Relational Operator8/1 -> Logical Operator2/3
  Divide/1 -> Gain6/1
  Gain4/1 -> Relational Operator8/1
  Numerator/1 -> Divide/1
  Relational Operator5/1 -> Logical Operator1/3
  Demux/3 -> [R31]
  Demux/4 -> [R12]
  Relational Operator9/1 -> Logical Operator3/1
  [R22] -> Relational Operator4/2
  [R22] -> Relational Operator9/2
  [R33] -> Relational Operator5/2
  Relational Operator2/1 -> Logical Operator/3
  Relational Operator4/1 -> Logical Operator1/2
  Demux/6 -> [R32]
  [R22] -> Relational Operator/1
  [R11] -> Relational Operator4/1
  [R11] -> Relational Operator5/1
  Logical Operator/1 -> [C0]
  [R33] -> Gain/1
  Denominator^2/1 -> Sqrt/1
  Relational Operator10/1 -> Logical Operator3/2
  [R33] -> Relational Operator9/1
  Gain5/1 -> Relational Operator10/1
  Gain3/1 -> Relational Operator3/1
  [R12] -> Add5/1
  [R21] -> Add7/2
  [R21] -> Add3/2
  Constant14/1 -> C1 sw/1
  [N0] -> Numerator/2
  Add7/1 -> Mux2/2
  Mux1/1 -> [N1]
  [N3] -> Numerator/5
  Constant17/1 -> C3 sw/3
  [R12] -> Add7/1
  Constant6/1 -> Divide1/1
  C2 sw/1 -> C1 sw/3
  [N0] -> Numerator/6
  Divide2/1 -> Mux5/2
  Divide1/1 -> Mux4/1
  Add/1 -> Mux4/4, Mux4/3, Mux4/2, Divide1/2
  [R23] -> Add1/1
  Switch/1 -> Product8/1
  Constant/1 -> Switch/3
  Constant18/1 -> Switch/1
  Compare To Zero/1 -> Switch/2
  Selector/1 -> Compare To Zero/1
  Reshape1/1 -> quat/1
  Product8/1 -> Reshape1/1
